simulink library "pathFollowingControllerManta_cl"  (R2020a)
settings: Solver=VariableStepAuto  StartTime=0.0  StopTime=10.0  RelTol=1e-3
undefined symbols (not defined in the file or in its folder): env, FLIGHTCONTROLLER, fltCtrl, hiLvlCtrl, initializeBussesFromBlock, vhcl
libraries: simulink x7, filteredPIDController_ul x2, velocityAngle_ul x2, filteredPIDControllerAWGS_ul x1, stopwatch_ul x1, courseFollowManta_cl x1, ctrlAllocMatrix_cl x1, eulAng2RotMat_ul x1, angleBtw2Vecs_ul x1, vrlib x1, alphaBeta_ul x1, gnd2TanRotation_ul x1
settings Model: Creator=jldanie5  LastModifiedBy=John Jr
settings DataIOCC: ReturnWorkspaceOutputs=off
settings DebuggingCC: ArithmeticOperatorsInVariantConditions=warning
settings SFSimCC: CustomCodeUndefinedFunction=UseInterfaceOnly

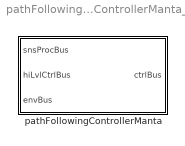
== system pathFollowingControllerManta_cl ==
  pathFollowingControllerManta : Subsystem  LoadFcn=initializeBussesFromBlock(gcb)  InitFcn=initializeBussesFromBlock(gcb)  StartFcn=initializeBussesFromBlock(gcb)  VariantControl=strcmpi(FLIGHTCONTROLLER,'pathFollowingControllerManta')  mask{initPosForInitSStar=vhcl.initPosVecGnd.Value, fluidDensity=env.water.density.Value, pathCtrl=fltCtrl, aeroStruct=vhcl.struct('OCT.aeroSurf')}
      mask prompts: initPosForInitSStar "Initial Position"; fluidDensity "Fluid Density"; pathCtrl "Controller"; aeroStruct "Aerodynamic Structure"
      settings: MinAlgLoopOccurrences=on
      mask DialogControl Container3 Prompt: courseFollow Params
      mask DialogControl Container4 Prompt: setpointToOutput Params

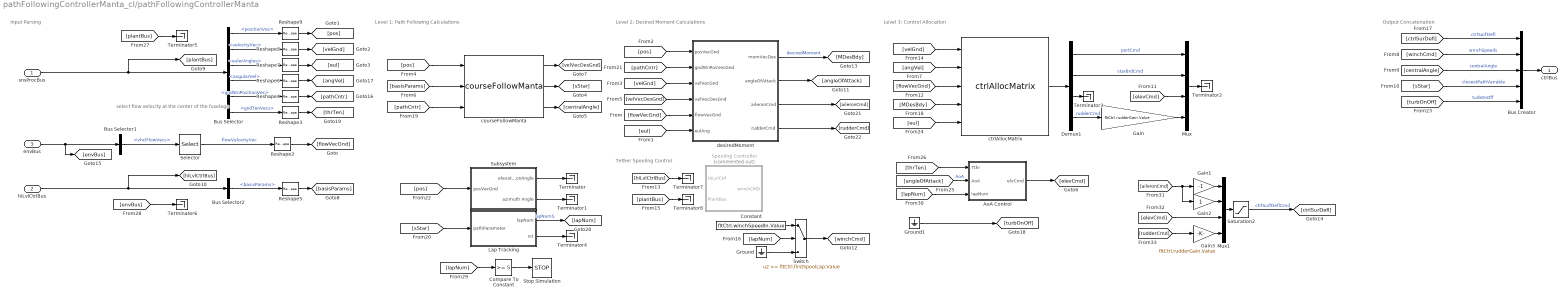
== system pathFollowingControllerManta_cl/pathFollowingControllerManta ==
  note: select flow velocity at the center of the fuselage
  note: Level 3: Control Allocation
  note: Output Concatenation
  note: Tether Spooling Control
  note: Level 2: Desired Moment Calculations
  note: Level 1: Path Following Calculations
  note: Input Parsing
  snsProcBus : Inport  OutDataTypeStr=Bus: sensorsProcessingBus
  hiLvlCtrlBus : Inport  Port=2  OutDataTypeStr=Bus: hiLvlCtrlBus
  envBus : Inport  Port=3  OutDataTypeStr=Bus: envBus
  AoA Control : Subsystem
  Bus Creator : BusCreator  Inputs=5  OutDataTypeStr=Bus: fltCtrlBus
      settings: InheritFromInputs=off
  Bus Selector : BusSelector  OutputSignals=positionVec,velocityVec,eulerAngles,angularVel,gndStnPositionVec,gndTenVecs
  Bus Selector1 : BusSelector  OutputSignals=vhclFlowVecs
  Bus Selector2 : BusSelector  OutputSignals=basisParams
  Compare To Constant : simulink/Logic and Bit Operations/Compare To Constant  relop=>=  const=5  OutDataTypeStr=boolean
  Constant : Constant  Value=fltCtrl.winchSpeedIn.Value
  Demux1 : Demux
  Gain : Gain  Gain=fltCtrl.rudderGain.Value
  Gain1 : Gain  Gain=-1
  Gain2 : Gain
  Gain3 : Gain  Gain=fltCtrl.rudderGain.Value
  Ground : Ground
  Ground1 : Ground
  Lap Tracking : Subsystem
  Mux : Mux
  Mux1 : Mux
  Reshape{1..3,5..9} (8 alike) : Reshape  OutputDimensionality=Column vector (2-D)
  Saturation2 : Saturate  UpperLimit=pathCtrl.controlSigMax.upperLimit.Value  LowerLimit=pathCtrl.controlSigMax.lowerLimit.Value
  Selector : Selector  NumberOfDimensions=2  InputPortWidth=3  IndexOptions=Select all,Index vector (dialog)  Indices=[1 3],5  OutputSizes=1,1
  "Spooling Controller " : Subsystem  Commented=on
  Stop Simulation : Stop
  Subsystem : Subsystem
  Switch : Switch  Threshold=fltCtrl.firstSpoolLap.Value
  Terminator{,1..8} (9 alike) : Terminator
  courseFollowManta : courseFollowManta_cl/courseFollowManta  SystemSampleTime=-1  Latency=0  AutoFrameSizeCalculation=off
  ctrlAllocMatrix : ctrlAllocMatrix_cl/ctrlAllocMatrix  aeroStruct=aeroStruct  fluidDensity=fluidDensity
  desiredMoment : Subsystem
  ctrlBus : Outport  OutDataTypeStr=Bus: fltCtrlBus  VectorParamsAs1DForOutWhenUnconnected=off
  wires:
  Bus Selector/6 -> Reshape3/1  "<gndTenVecs>"
  Reshape3/1 -> [thrTen]
  courseFollowManta/1 -> [velVecDesGnd]
  snsProcBus/1 -> Bus Selector/1, [plantBus]
  Bus Selector/2 -> Reshape8/1  "<velocityVec>"
  Bus Selector/1 -> Reshape9/1  "<positionVec>"
  Bus Selector/3 -> Reshape7/1  "<eulerAngles>"
  [pos] -> courseFollowManta/1
  Bus Creator/1 -> ctrlBus/1
  [winchCmd] -> Bus Creator/2  "winchSpeeds"
  courseFollowManta/2 -> [sStar]
  hiLvlCtrlBus/1 -> [hiLvlCtrlBus], Bus Selector2/1
  [centralAngle] -> Bus Creator/3  "centralAngle"
  [sStar] -> Bus Creator/4  "closestPathVariable"
  courseFollowManta/3 -> [centralAngle]
  desiredMoment/1(momVecDes) -> [MDesBdy]  "desiredMoment"
  Bus Selector/4 -> Reshape6/1  "<angularVel>"
  [angVel] -> ctrlAllocMatrix/2
  [velGnd] -> ctrlAllocMatrix/1
  [flowVecGnd] -> ctrlAllocMatrix/3
  Demux1/3 -> Terminator3/1
  Demux1/1 -> Mux/1  "portCmd"
  Demux1/2 -> Mux/2  "starBrdCmd"
  [MDesBdy] -> ctrlAllocMatrix/4
  [ctrlSurDefl] -> Bus Creator/1  "ctrlSurfDefl"
  Bus Selector2/1 -> Reshape5/1  "<basisParams>"
  Reshape5/1 -> [basisParams]
  Saturation2/1 -> [ctrlSurDefl]  "ctrlSurfDeflCmd"
  Reshape2/1 -> [flowVecGnd]
  Reshape6/1 -> [angVel]
  Reshape7/1 -> [eul]
  Reshape8/1 -> [velGnd]
  Reshape9/1 -> [pos]
  [eul] -> ctrlAllocMatrix/5
  Selector/1 -> Reshape2/1  "flowVelocityVec"
  envBus/1 -> [envBus], Bus Selector1/1
  Bus Selector1/1 -> Selector/1  "<vhclFlowVecs>"
  Reshape1/1 -> [pathCntr]
  Bus Selector/5 -> Reshape1/1  "<gndStnPositionVec>"
  [pathCntr] -> courseFollowManta/3
  [pos] -> desiredMoment/1(posVecGnd)
  [pathCntr] -> desiredMoment/2(gndStnPosVecGnd)
  [velGnd] -> desiredMoment/3(velVecGnd)
  [velVecDesGnd] -> desiredMoment/4(velVecDesGnd)
  [eul] -> desiredMoment/6(eulAng)
  [flowVecGnd] -> desiredMoment/5(flowVecGnd)
  [basisParams] -> courseFollowManta/2
  Demux1/4 -> Gain/1  "rudderCmd"
  [turbOnOff] -> Bus Creator/5  "turbOnOff"
  [pos] -> Subsystem/1(posVecGnd)
  Subsystem/1(elevationAngle) -> Terminator/1
  Subsystem/2(azimuth Angle) -> Terminator1/1
  [elevCmd] -> Mux/3
  desiredMoment/2(angleOfAttack) -> [angleOfAttack]
  Ground1/1 -> [turbOnOff]
  [thrTen] -> AoA Control/1(Tthr)
  [angleOfAttack] -> AoA Control/2(AoA)  "AoA"
  AoA Control/1(elvCmd) -> [elevCmd]
  [sStar] -> Lap Tracking/1(pathParameter)
  Lap Tracking/2(rst) -> Terminator4/1
  Lap Tracking/1(lapNum) -> [lapNum]  "lapNumS"
  [plantBus] -> Terminator5/1
  [envBus] -> Terminator6/1
  [hiLvlCtrlBus] -> Terminator7/1
  [plantBus] -> Terminator8/1
  Switch/1 -> [winchCmd]
  [lapNum] -> Switch/2
  Constant/1 -> Switch/1
  Ground/1 -> Switch/3
  [lapNum] -> Compare To Constant/1
  Compare To Constant/1 -> Stop Simulation/1
  [lapNum] -> AoA Control/3(lapNum)
  desiredMoment/3(aileronCmd) -> [aileronCmd]
  [aileronCmd] -> Gain2/1, Gain1/1
  Gain1/1 -> Mux1/1
  Gain2/1 -> Mux1/2
  [elevCmd] -> Mux1/3
  Gain/1 -> Mux/4
  Mux1/1 -> Saturation2/1
  desiredMoment/4(rudderCmd) -> [rudderCmd]
  [rudderCmd] -> Gain3/1
  Gain3/1 -> Mux1/4
  ctrlAllocMatrix/1 -> Demux1/1
  Mux/1 -> Terminator2/1

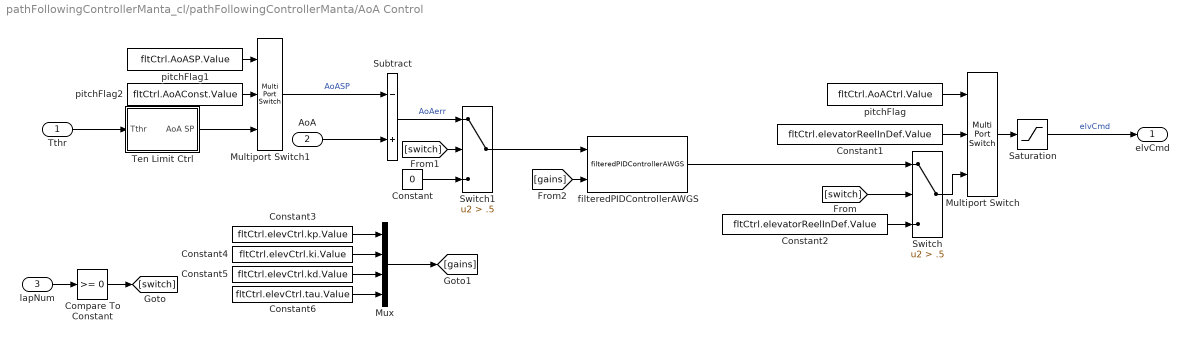
== system pathFollowingControllerManta_cl/pathFollowingControllerManta/AoA Control ==
  Tthr : Inport
  AoA : Inport  Port=2
  lapNum : Inport  Port=3
  Compare To Constant : simulink/Logic and Bit Operations/Compare To Constant  relop=>=  const=0  OutDataTypeStr=boolean
  Constant : Constant  Value=0
  Constant1 : Constant  Value=fltCtrl.elevatorReelInDef.Value
  Constant2 : Constant  Value=fltCtrl.elevatorReelInDef.Value
  Constant3 : Constant  Value=fltCtrl.elevCtrl.kp.Value
  Constant4 : Constant  Value=fltCtrl.elevCtrl.ki.Value
  Constant5 : Constant  Value=fltCtrl.elevCtrl.kd.Value
  Constant6 : Constant  Value=fltCtrl.elevCtrl.tau.Value
  Multiport Switch : MultiPortSwitch  DataPortOrder=Specify indices  Inputs=2  DataPortIndices={0,1}
  Multiport Switch1 : MultiPortSwitch  DataPortOrder=Specify indices  Inputs=2  DataPortIndices={0,1}
  Mux : Mux
  Saturation : Saturate  UpperLimit=fltCtrl.elevCtrlMax.upperLimit.Value  LowerLimit=fltCtrl.elevCtrlMax.lowerLimit.Value
  Subtract : Sum  Inputs=-+
  Switch : Switch  Criteria=u2 > Threshold  Threshold=.5
  Switch1 : Switch  Criteria=u2 > Threshold  Threshold=.5
  Ten Limit Ctrl : Subsystem
  filteredPIDControllerAWGS : filteredPIDControllerAWGS_ul/filteredPIDControllerAWGS  cmax=fltCtrl.elevCtrlMax.upperLimit.Value  cmin=fltCtrl.elevCtrlMax.lowerLimit.Value
  pitchFlag : Constant  Value=fltCtrl.AoACtrl.Value
  pitchFlag1 : Constant  Value=fltCtrl.AoASP.Value
  pitchFlag2 : Constant  Value=fltCtrl.AoAConst.Value
  elvCmd : Outport
  wires:
  AoA/1 -> Subtract/2
  Tthr/1 -> Ten Limit Ctrl/1(Tthr)
  Constant1/1 -> Multiport Switch/2
  pitchFlag2/1 -> Multiport Switch1/2
  pitchFlag/1 -> Multiport Switch/1
  pitchFlag1/1 -> Multiport Switch1/1
  Multiport Switch1/1 -> Subtract/1  "AoASP"
  Ten Limit Ctrl/1(AoA SP) -> Multiport Switch1/3
  Multiport Switch/1 -> Saturation/1
  Constant2/1 -> Switch/3
  Saturation/1 -> elvCmd/1  "elvCmd"
  lapNum/1 -> Compare To Constant/1
  Compare To Constant/1 -> [switch]
  [switch] -> Switch/2
  Subtract/1 -> Switch1/1  "AoAerr"
  [switch] -> Switch1/2
  Constant/1 -> Switch1/3
  Switch/1 -> Multiport Switch/3
  Switch1/1 -> filteredPIDControllerAWGS/1
  filteredPIDControllerAWGS/1 -> Switch/1
  [gains] -> filteredPIDControllerAWGS/2
  Mux/1 -> [gains]
  Constant3/1 -> Mux/1
  Constant4/1 -> Mux/2
  Constant5/1 -> Mux/3
  Constant6/1 -> Mux/4

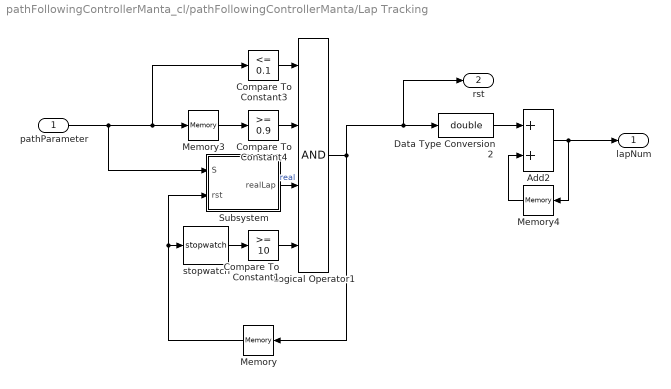
== system pathFollowingControllerManta_cl/pathFollowingControllerManta/Lap Tracking ==
  pathParameter : Inport
  Add2 : Sum
  Compare To Constant1 : simulink/Logic and Bit Operations/Compare To Constant  relop=>=  const=10  OutDataTypeStr=boolean
  Compare To Constant3 : simulink/Logic and Bit Operations/Compare To Constant  relop=<=  const=0.1  OutDataTypeStr=boolean
  Compare To Constant4 : simulink/Logic and Bit Operations/Compare To Constant  relop=>=  const=0.9  OutDataTypeStr=boolean
  Data Type Conversion2 : DataTypeConversion  OutDataTypeStr=double
  Logical Operator1 : Logic  Inputs=4  AllPortsSameDT=off  OutDataTypeStr=boolean
  Memory : Memory  InitialCondition=false
  Memory3 : Memory
  Memory4 : Memory
  Subsystem : Subsystem
  stopwatch : stopwatch_ul/stopwatch  SystemSampleTime=-1  Latency=0  AutoFrameSizeCalculation=off
  lapNum : Outport  VectorParamsAs1DForOutWhenUnconnected=off
  rst : Outport  Port=2  VectorParamsAs1DForOutWhenUnconnected=off
  wires:
  Compare To Constant3/1 -> Logical Operator1/1
  Memory3/1 -> Compare To Constant4/1
  Data Type Conversion2/1 -> Add2/1
  Logical Operator1/1 -> rst/1, Data Type Conversion2/1, Memory/1
  Memory4/1 -> Add2/2
  Add2/1 -> lapNum/1, Memory4/1
  Compare To Constant4/1 -> Logical Operator1/2
  pathParameter/1 -> Subsystem/1(S), Compare To Constant3/1, Memory3/1
  stopwatch/1 -> Compare To Constant1/1
  Memory/1 -> Subsystem/2(rst), stopwatch/1
  Compare To Constant1/1 -> Logical Operator1/4
  Subsystem/1(realLap) -> Logical Operator1/3  "real"

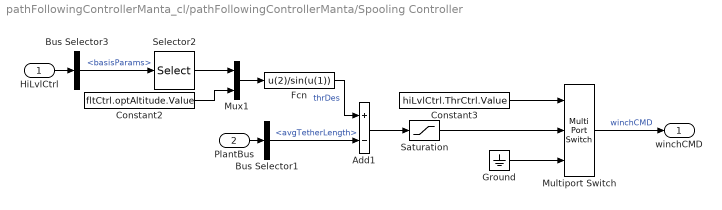
== system pathFollowingControllerManta_cl/pathFollowingControllerManta/Spooling Controller  ==
  HiLvlCtrl : Inport
  PlantBus : Inport  Port=2
  Add1 : Sum  Inputs=+-
  Bus Selector1 : BusSelector  OutputSignals=avgTetherLength
  Bus Selector3 : BusSelector  OutputSignals=basisParams
  Constant2 : Constant  Value=fltCtrl.optAltitude.Value
  Constant3 : Constant  Value=hiLvlCtrl.ThrCtrl.Value
  Fcn : Fcn  Expr=u(2)/sin(u(1))
  Ground : Ground
  Multiport Switch : MultiPortSwitch  DataPortOrder=Specify indices  Inputs=2  DataPortIndices={0,1}
  Mux1 : Mux  Inputs=2
  Saturation : Saturate  UpperLimit=.25  LowerLimit=-.25
  Selector2 : Selector  InputPortWidth=5  IndexOptions=Index vector (dialog)  Indices=3  OutputSizes=1
  winchCMD : Outport
  wires:
  Bus Selector3/1 -> Selector2/1  "<basisParams>"
  Mux1/1 -> Fcn/1
  Bus Selector1/1 -> Add1/2  "<avgTetherLength>"
  Constant2/1 -> Mux1/2
  Add1/1 -> Saturation/1
  Fcn/1 -> Add1/1  "thrDes"
  Selector2/1 -> Mux1/1
  Multiport Switch/1 -> winchCMD/1  "winchCMD"
  HiLvlCtrl/1 -> Bus Selector3/1
  Ground/1 -> Multiport Switch/3
  Saturation/1 -> Multiport Switch/2
  Constant3/1 -> Multiport Switch/1
  PlantBus/1 -> Bus Selector1/1

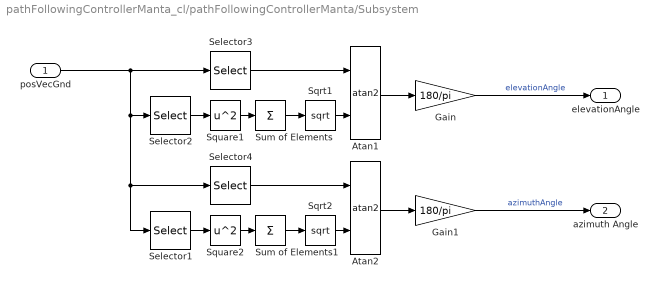
== system pathFollowingControllerManta_cl/pathFollowingControllerManta/Subsystem ==
  posVecGnd : Inport
  Atan1 : Trigonometry  Operator=atan2
  Atan2 : Trigonometry  Operator=atan2
  Gain : Gain  Gain=180/pi
  Gain1 : Gain  Gain=180/pi
  Selector1 : Selector  InputPortWidth=3  IndexOptions=Index vector (dialog)  Indices=1  OutputSizes=1
  Selector2 : Selector  InputPortWidth=3  IndexOptions=Index vector (dialog)  Indices=[1 2]  OutputSizes=1
  Selector3 : Selector  InputPortWidth=3  IndexOptions=Index vector (dialog)  Indices=3  OutputSizes=1
  Selector4 : Selector  InputPortWidth=3  IndexOptions=Index vector (dialog)  Indices=2  OutputSizes=1
  Sqrt1 : Sqrt  SaturateOnIntegerOverflow=on
  Sqrt2 : Sqrt  SaturateOnIntegerOverflow=on
  Square1 : Math  Operator=square  SignedPower=on  SaturateOnIntegerOverflow=on
  Square2 : Math  Operator=square  SignedPower=on  SaturateOnIntegerOverflow=on
  Sum of Elements : Sum  Inputs=+
  Sum of Elements1 : Sum  Inputs=+
  elevationAngle : Outport
  azimuth Angle : Outport  Port=2
  wires:
  Sqrt1/1 -> Atan1/2
  Square1/1 -> Sum of Elements/1
  Selector3/1 -> Atan1/1
  Sum of Elements/1 -> Sqrt1/1
  Atan1/1 -> Gain/1
  Selector2/1 -> Square1/1
  Gain/1 -> elevationAngle/1  "elevationAngle"
  Atan2/1 -> Gain1/1
  Square2/1 -> Sum of Elements1/1
  Sum of Elements1/1 -> Sqrt2/1
  Selector1/1 -> Square2/1
  posVecGnd/1 -> Selector1/1, Selector4/1, Selector2/1, Selector3/1
  Sqrt2/1 -> Atan2/2
  Selector4/1 -> Atan2/1
  Gain1/1 -> azimuth Angle/1  "azimuthAngle"

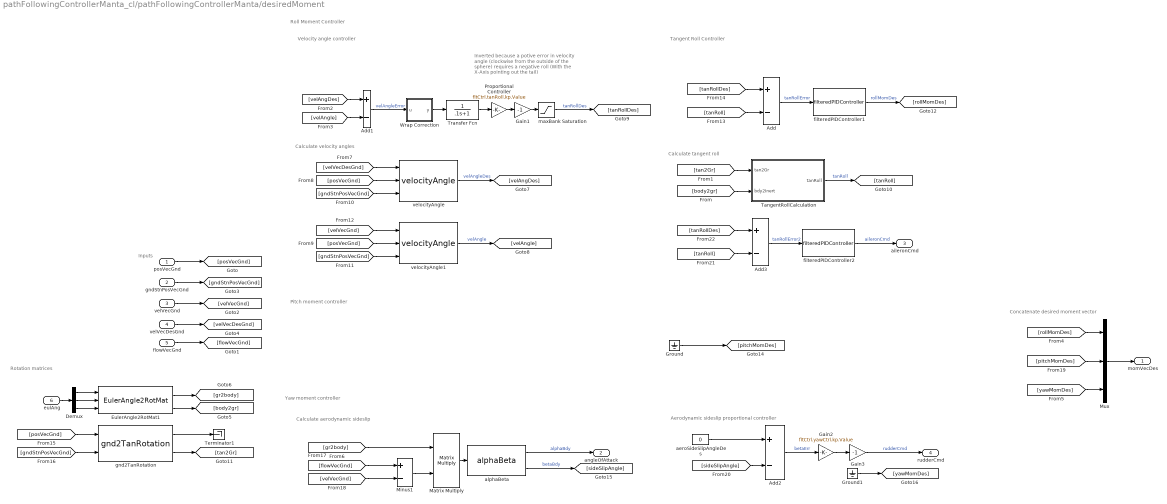
== system pathFollowingControllerManta_cl/pathFollowingControllerManta/desiredMoment ==
  note: Yaw moment controller
  note: Pitch moment controller
  note: Inverted because a potive error
      | in velocity angle (clockwise from the
      | outside of the sphere) requires a negative
      | roll (With the X-Axis pointing out the tail)
  note: Velocity angle controller
  note: Inputs
  note: Rotation matrices
  note: Calculate velocity angles
  note: Calculate tangent roll
  note: Tangent Roll Controller
  note: Concatenate desired moment vector
  note: Roll Moment Controller
  note: Aerodynamic sideslip proportional controller
  note: Calculate aerodynamic sideslip
  posVecGnd : Inport
  gndStnPosVecGnd : Inport  Port=2
  velVecGnd : Inport  Port=3
  velVecDesGnd : Inport  Port=4
  flowVecGnd : Inport  Port=5
  eulAng : Inport  Port=6
  Add{,1..3} (4 alike) : Sum  Inputs=+-
  Demux : Demux  Outputs=3
  EulerAngle2RotMat1 : eulAng2RotMat_ul/EulerAngle2RotMat  SystemSampleTime=-1  Latency=0  AutoFrameSizeCalculation=off
  Gain1 : Gain  Gain=-1
  Gain2 : Gain  Gain=fltCtrl.yawCtrl.kp.Value
  Gain3 : Gain  Gain=-1
  Ground : Ground
  Ground1 : Ground
  Matrix Multiply : Product  Multiplication=Matrix(*)
  Minus1 : Sum  Inputs=+-
  Mux : Mux  Inputs=3
  Proportional Controller : Gain  Gain=fltCtrl.tanRoll.kp.Value
  TangentRollCalculation : Subsystem
  Terminator1 : Terminator
  Transfer Fcn : TransferFcn  Denominator=[.1 1]
  Wrap Correction : Subsystem
  aeroSideSlipAngleDes : Constant  Value=0
  alphaBeta : alphaBeta_ul/alphaBeta  SystemSampleTime=-1  Latency=0  AutoFrameSizeCalculation=off
  filteredPIDController1 : filteredPIDController_ul/filteredPIDController  kp=pathCtrl.rollMoment.kp.Value  ki=0  kd=pathCtrl.rollMoment.kd.Value  Value=pathCtrl.rollMoment.tau.Value  externalReset=none
  filteredPIDController2 : filteredPIDController_ul/filteredPIDController  kp=fltCtrl.rollCtrl.kp.Value  ki=fltCtrl.rollCtrl.ki.Value  kd=fltCtrl.rollCtrl.kd.Value  Value=fltCtrl.rollCtrl.tau.Value  externalReset=none
  gnd2TanRotation : gnd2TanRotation_ul/gnd2TanRotation  SystemSampleTime=-1  Latency=0  AutoFrameSizeCalculation=off
  maxBank Saturation : Saturate  UpperLimit=pathCtrl.maxBank.upperLimit.Value  LowerLimit=pathCtrl.maxBank.lowerLimit.Value
  velocityAngle : velocityAngle_ul/velocityAngle  SystemSampleTime=-1  Latency=0  AutoFrameSizeCalculation=off
  velocityAngle1 : velocityAngle_ul/velocityAngle  SystemSampleTime=-1  Latency=0  AutoFrameSizeCalculation=off
  momVecDes : Outport  VectorParamsAs1DForOutWhenUnconnected=off
  angleOfAttack : Outport  Port=2  VectorParamsAs1DForOutWhenUnconnected=off
  aileronCmd : Outport  Port=3  VectorParamsAs1DForOutWhenUnconnected=off
  rudderCmd : Outport  Port=4  VectorParamsAs1DForOutWhenUnconnected=off
  wires:
  [sideSlipAngle] -> Add2/2
  [yawMomDes] -> Mux/3
  [rollMomDes] -> Mux/1
  gnd2TanRotation/1 -> Terminator1/1
  gnd2TanRotation/2 -> [tan2Gr]
  [gndStnPosVecGnd] -> gnd2TanRotation/2
  [posVecGnd] -> gnd2TanRotation/1
  [tanRollDes] -> Add/1
  [tanRoll] -> Add/2
  [velVecGnd] -> velocityAngle1/1
  [gndStnPosVecGnd] -> velocityAngle1/3
  [gndStnPosVecGnd] -> velocityAngle/3
  [posVecGnd] -> velocityAngle1/2
  [posVecGnd] -> velocityAngle/2
  [velVecDesGnd] -> velocityAngle/1
  [velAngle] -> Add1/2
  [velAngDes] -> Add1/1
  velocityAngle1/1 -> [velAngle]  "velAngle"
  velocityAngle/1 -> [velAngDes]  "velAngleDes"
  velVecDesGnd/1 -> [velVecDesGnd]
  gndStnPosVecGnd/1 -> [gndStnPosVecGnd]
  [pitchMomDes] -> Mux/2
  alphaBeta/1 -> angleOfAttack/1  "alphaBdy"
  Mux/1 -> momVecDes/1
  aeroSideSlipAngleDes/1 -> Add2/1
  Add2/1 -> Gain2/1  "betaErr"
  alphaBeta/2 -> [sideSlipAngle]  "betaBdy"
  Matrix Multiply/1 -> alphaBeta/1
  [gr2body] -> Matrix Multiply/1
  [body2gr] -> TangentRollCalculation/2(bdy2Inert)
  EulerAngle2RotMat1/1 -> [gr2body]
  EulerAngle2RotMat1/2 -> [body2gr]
  Demux/2 -> EulerAngle2RotMat1/2
  Demux/1 -> EulerAngle2RotMat1/1
  Demux/3 -> EulerAngle2RotMat1/3
  eulAng/1 -> Demux/1
  [flowVecGnd] -> Minus1/1
  [velVecGnd] -> Minus1/2
  Minus1/1 -> Matrix Multiply/2
  Gain2/1 -> Gain3/1
  filteredPIDController1/1 -> [rollMomDes]  "rollMomDes"
  TangentRollCalculation/1(tanRoll) -> [tanRoll]  "tanRoll"
  [tan2Gr] -> TangentRollCalculation/1(tan2Gr)
  flowVecGnd/1 -> [flowVecGnd]
  Add1/1 -> Wrap Correction/1(u)  "velAngleError"
  maxBank Saturation/1 -> [tanRollDes]  "tanRollDes"
  Gain1/1 -> maxBank Saturation/1
  Proportional Controller/1 -> Gain1/1
  Add/1 -> filteredPIDController1/1  "tanRollError"
  velVecGnd/1 -> [velVecGnd]
  posVecGnd/1 -> [posVecGnd]
  Ground/1 -> [pitchMomDes]
  Wrap Correction/1(y) -> Transfer Fcn/1
  Transfer Fcn/1 -> Proportional Controller/1
  Add3/1 -> filteredPIDController2/1  "tanRollError2"
  [tanRoll] -> Add3/2
  [tanRollDes] -> Add3/1
  filteredPIDController2/1 -> aileronCmd/1  "aileronCmd"
  Ground1/1 -> [yawMomDes]
  Gain3/1 -> rudderCmd/1  "rudderCmd"

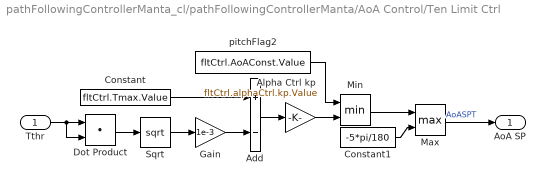
== system pathFollowingControllerManta_cl/pathFollowingControllerManta/AoA Control/Ten Limit Ctrl ==
  Tthr : Inport
  Add : Sum  Inputs=+-
  Alpha Ctrl kp : Gain  Gain=fltCtrl.alphaCtrl.kp.Value
  Constant : Constant  Value=fltCtrl.Tmax.Value
  Constant1 : Constant  Value=-5*pi/180
  Dot Product : DotProduct  InputSameDT=on  OutDataTypeStr=Inherit: Inherit via internal rule
  Gain : Gain  Gain=1e-3
  Max : MinMax  Function=max  Inputs=2
  Min : MinMax  Inputs=2
  Sqrt : Sqrt  SaturateOnIntegerOverflow=on
  pitchFlag2 : Constant  Value=fltCtrl.AoAConst.Value
  AoA SP : Outport
  wires:
  Tthr/1 -> Dot Product/2, Dot Product/1
  Dot Product/1 -> Sqrt/1
  Constant/1 -> Add/1
  Sqrt/1 -> Gain/1
  Add/1 -> Alpha Ctrl kp/1
  Gain/1 -> Add/2
  Alpha Ctrl kp/1 -> Min/2
  pitchFlag2/1 -> Min/1
  Min/1 -> Max/1
  Max/1 -> AoA SP/1  "AoASPT"
  Constant1/1 -> Max/2

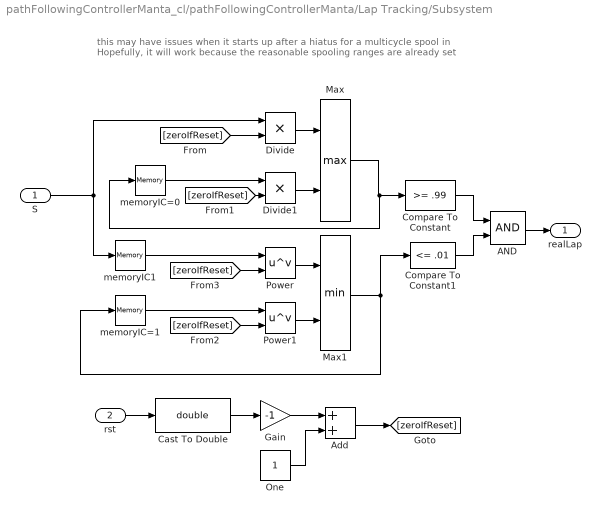
== system pathFollowingControllerManta_cl/pathFollowingControllerManta/Lap Tracking/Subsystem ==
  note: this may have issues when it starts up after a hiatus for a multicycle spool in
      | Hopefully, it will work because the reasonable spooling ranges are already set
  S : Inport
  rst : Inport  Port=2
  AND : Logic  AllPortsSameDT=off  OutDataTypeStr=boolean
  Add : Sum
  Cast To Double : DataTypeConversion  OutDataTypeStr=double
  Compare To Constant : simulink/Logic and Bit Operations/Compare To Constant  relop=>=  const=.99  OutDataTypeStr=boolean
  Compare To Constant1 : simulink/Logic and Bit Operations/Compare To Constant  relop=<=  const=.01  OutDataTypeStr=boolean
  Divide : Product  Inputs=**
  Divide1 : Product  Inputs=**
  Gain : Gain  Gain=-1
  Max : MinMax  Function=max  Inputs=2
  Max1 : MinMax  Inputs=2
  One : Constant  OutDataTypeStr=Inherit: Inherit via back propagation
  Power : Math  Operator=pow  SaturateOnIntegerOverflow=on
  Power1 : Math  Operator=pow  SaturateOnIntegerOverflow=on
  memoryIC1 : Memory  InitialCondition=1
  memoryIC=0 : Memory
  memoryIC=1 : Memory  InitialCondition=1
  realLap : Outport
  wires:
  Max1/1 -> Compare To Constant1/1, memoryIC=1/1
  rst/1 -> Cast To Double/1
  S/1 -> Divide/1, memoryIC1/1
  Gain/1 -> Add/1
  Add/1 -> [zeroIfReset]
  One/1 -> Add/2
  Divide/1 -> Max/1
  Max/1 -> memoryIC=0/1, Compare To Constant/1
  Power/1 -> Max1/1
  Power1/1 -> Max1/2
  Cast To Double/1 -> Gain/1
  Compare To Constant/1 -> AND/1
  Compare To Constant1/1 -> AND/2
  AND/1 -> realLap/1
  [zeroIfReset] -> Divide/2
  [zeroIfReset] -> Power/2
  [zeroIfReset] -> Divide1/2
  Divide1/1 -> Max/2
  memoryIC=0/1 -> Divide1/1
  [zeroIfReset] -> Power1/2
  memoryIC=1/1 -> Power1/1
  memoryIC1/1 -> Power/1

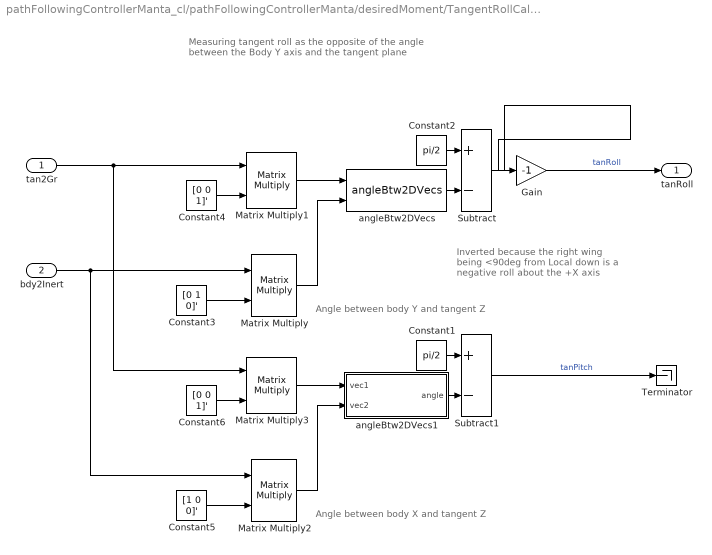
== system pathFollowingControllerManta_cl/pathFollowingControllerManta/desiredMoment/TangentRollCalculation ==
  note: Angle between body X and tangent Z
  note: Inverted because the right wing
      | being <90deg from Local down
      | is a negative roll about the +X axis
  note: Angle between body Y and tangent Z
  note: Measuring tangent roll as the opposite
      | of the angle between the Body Y axis
      | and the tangent plane
  tan2Gr : Inport
  bdy2Inert : Inport  Port=2
  Constant1 : Constant  Value=pi/2
  Constant2 : Constant  Value=pi/2
  Constant3 : Constant  Value=[0 1 0]'
  Constant4 : Constant  Value=[0 0 1]'
  Constant5 : Constant  Value=[1 0 0]'
  Constant6 : Constant  Value=[0 0 1]'
  Gain : Gain  Gain=-1
  Matrix Multiply{,1..3} (4 alike) : Product  Multiplication=Matrix(*)
  Subtract : Sum  Inputs=+-
  Subtract1 : Sum  Inputs=+-
  Terminator : Terminator
  angleBtw2DVecs : angleBtw2Vecs_ul/angleBtw2DVecs  SystemSampleTime=-1  Latency=0  AutoFrameSizeCalculation=off
  angleBtw2DVecs1 : Subsystem
  tanRoll : Outport  VectorParamsAs1DForOutWhenUnconnected=off
  wires:
  Constant5/1 -> Matrix Multiply2/2
  angleBtw2DVecs1/1(angle) -> Subtract1/2
  Constant1/1 -> Subtract1/1
  Matrix Multiply3/1 -> angleBtw2DVecs1/1(vec1)
  Constant6/1 -> Matrix Multiply3/2
  Matrix Multiply2/1 -> angleBtw2DVecs1/2(vec2)
  tan2Gr/1 -> Matrix Multiply1/1, Matrix Multiply3/1
  Subtract1/1 -> Terminator/1  "tanPitch"
  bdy2Inert/1 -> Matrix Multiply/1, Matrix Multiply2/1
  Gain/1 -> tanRoll/1  "tanRoll"
  Matrix Multiply/1 -> angleBtw2DVecs/2
  Constant4/1 -> Matrix Multiply1/2
  Matrix Multiply1/1 -> angleBtw2DVecs/1
  Constant2/1 -> Subtract/1
  angleBtw2DVecs/1 -> Subtract/2
  Constant3/1 -> Matrix Multiply/2
  Subtract/1 -> Gain/1

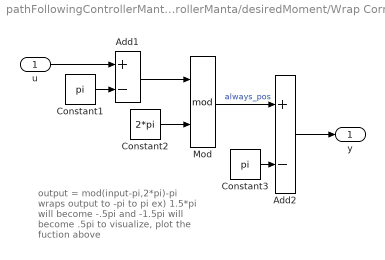
== system pathFollowingControllerManta_cl/pathFollowingControllerManta/desiredMoment/Wrap Correction ==
  note: output = mod(input-pi,2*pi)-pi
      | wraps output to -pi to pi
      |
      | ex) 1.5*pi will become -.5pi
      | 	and -1.5pi will become .5pi
      |
      | to visualize, plot the fuction above
  u : Inport
  Add1 : Sum  Inputs=+-
  Add2 : Sum  Inputs=+-
  Constant1 : Constant  Value=pi
  Constant2 : Constant  Value=2*pi
  Constant3 : Constant  Value=pi
  Mod : Math  Operator=mod  SignedPower=on  SaturateOnIntegerOverflow=on
  y : Outport  VectorParamsAs1DForOutWhenUnconnected=off
  wires:
  Add2/1 -> y/1
  Constant3/1 -> Add2/2
  Mod/1 -> Add2/1  "always_pos"
  Constant2/1 -> Mod/2
  Add1/1 -> Mod/1
  Constant1/1 -> Add1/2
  u/1 -> Add1/1

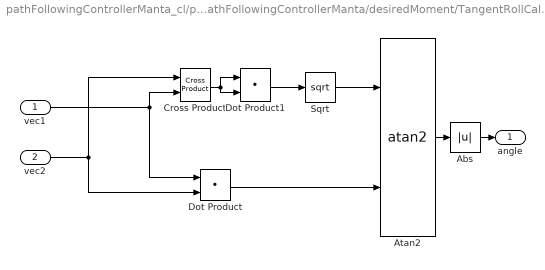
== system pathFollowingControllerManta_cl/pathFollowingControllerManta/desiredMoment/TangentRollCalculation/angleBtw2DVecs1 ==
  vec1 : Inport
  vec2 : Inport  Port=2
  Abs : Abs
  Atan2 : Trigonometry  Operator=atan2
  Cross Product : vrlib/Utilities/Cross Product
      settings: SourceProductBaseCode=VR
  Dot Product : DotProduct  InputSameDT=on  OutDataTypeStr=Inherit: Inherit via internal rule
  Dot Product1 : DotProduct  InputSameDT=on  OutDataTypeStr=Inherit: Inherit via internal rule
  Sqrt : Sqrt  SaturateOnIntegerOverflow=on
  angle : Outport  VectorParamsAs1DForOutWhenUnconnected=off
  wires:
  Sqrt/1 -> Atan2/1
  Dot Product1/1 -> Sqrt/1
  Abs/1 -> angle/1
  Dot Product/1 -> Atan2/2
  Cross Product/1 -> Dot Product1/2, Dot Product1/1
  vec2/1 -> Dot Product/2, Cross Product/1
  vec1/1 -> Cross Product/2, Dot Product/1
  Atan2/1 -> Abs/1
